simulink model "Lezione3model"  (R2022b)
settings: Solver=VariableStepAuto  StartTime=0.0  StopTime=10.0  RelTol=1e-3
undefined symbols (not defined in the file or in its folder): H
settings Model: Creator=giov_russo  LastModifiedBy=giov_russo

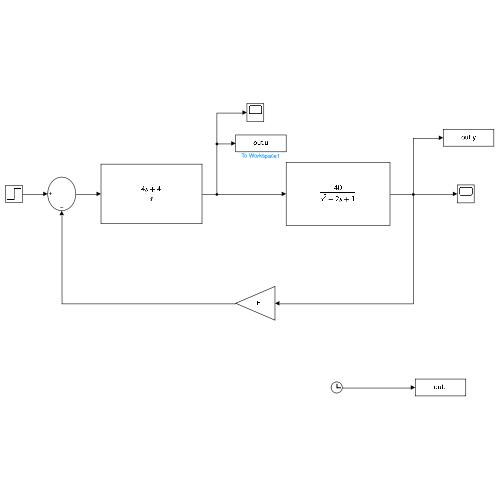
[thumbnail: Simulink's stored preview of the top-level diagram]
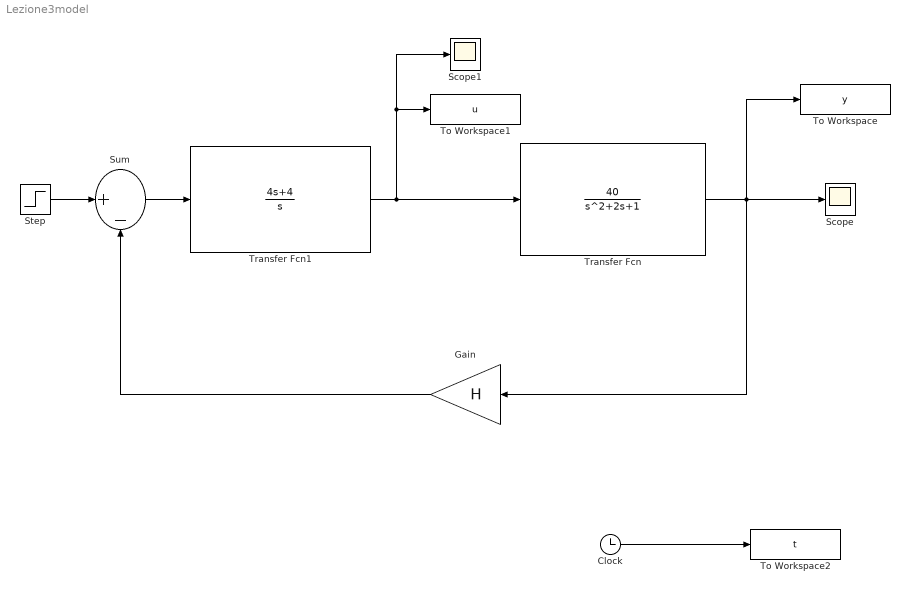
== system Lezione3model ==
  Clock : Clock
  Gain : Gain  Gain=H
  Scope : Scope
  Scope1 : Scope
  Step : Step  Time=0  SampleTime=0
  Sum : Sum  Inputs=|+-
  To Workspace : ToWorkspace  VariableName=y  SampleTime=-1
  To Workspace1 : ToWorkspace  VariableName=u  SampleTime=-1
  To Workspace2 : ToWorkspace  VariableName=t  SampleTime=-1
  Transfer Fcn : TransferFcn  Numerator=[40]
  Transfer Fcn1 : TransferFcn  Numerator=[4 4]  Denominator=[1 0]
  wires:
  Transfer Fcn1/1 -> Scope1/1, To Workspace1/1, Transfer Fcn/1
  Transfer Fcn/1 -> To Workspace/1, Scope/1, Gain/1
  Sum/1 -> Transfer Fcn1/1
  Gain/1 -> Sum/2
  Step/1 -> Sum/1
  Clock/1 -> To Workspace2/1
